simulink model "Huginn"  (R2024b)
settings: Solver=FixedStepAuto  StartTime=0.0  StopTime=525  FixedStep=0.1  RelTol=1e-3
model workspace (MAT data in the model file):
  N_P0 = 3
  fuel_map = [8.33e-06 8.33e-06 8.33e-06 8.33e-06 8.33e-06 8.33e-06 8.33e-06 8.33e-06 8.33e-06 8.33e-06 8.33e-06 8.33e-06 ... (2082 elements, 1041x2)]
  rpm_bp = [0 10 20 30 40 50 60 70 80 90 100 110 ... (671 elements, 671x1)]
  rpm_bp_fuel = [1200 1210 1220 1230 1240 1250 1260 1270 1280 1290 1300 1310 ... (1041 elements, 1041x1)]
  throttle_bp = [0 10 20 30 40 50 60 70 80 90 100]
  throttle_bp_fuel = [0; 1]
  torque_bp = [0.332105118453 0.337426322834 0.342845115066 0.348363542915 0.353983594259 0.359707194633 0.36553620448 0.371483133692 0.377549913828 0.383738457661 0.390050655328 0.396488370473 ... (901 elements, 901x1)]
  torque_map = [0 0 0 0 0 0 0 0 0 0 0 0 ... (7381 elements, 671x11)]
values from neighbouring files (symbols this model uses):
  rpm_fine = [1200 1210 1220 1230 1240 1250 1260 1270 1280 1290 1300 1310 ... (1041 elements, 1041x1)]    [optimised workspace.mat]    (also in run_before_huginn.m = (min(rpm_bp) : 10 : max(rpm_bp))')
  throttle_fine = [0 1]    [optimised workspace.mat]    (also in run_before_huginn.m = (min(throttle_bp) : 1 : max(throttle_bp))')
  throttle_profile = [14.9858312924 0 60 60 60 0.55631746946 8.17065947955 1.9881415447 9.75633320207 0.0428601079869 58.2417871472 60 ... (25 elements, 1x25)]    [Optimised_fuel_2.mat]    (also in optimised workspace.mat = [65.5401746966 57.4724229506 57.2057862197 67.539022656 57.9; other optmised.mat)
undefined symbols (not defined in the file or in its folder): DiscIntNeverNeededParam, dspblkCoreblockFVToolHelper, gcbh
(part 2 of 2)

== matlab function Huginn/Gear ==
  data: rpm input; rpm_out output; gear input; hold_timer input; g1 input; g2 input; g3 input; g4 input; up input; dn input; gear_out output; hold_out output; check output
function [rpm_out, gear_out, hold_out, check] = GearChange(rpm, gear, hold_timer, g1, g2, g3, g4, up, dn)
    ratios     = [g1, g2, g3, g4];
    num_gears  = numel(ratios);
    hysteresis = 0;   % increased from 150
    min_hold   = 20;
    check = 0; % 5 seconds at 0.1s timestep — increased from 20
    
    if hold_timer > 0
        rpm_out  = rpm;
        gear_out = double(gear);
        hold_out = hold_timer - 1;
    elseif rpm < (dn - hysteresis) && gear > 1
        rpm_out  = (ratios(gear-1) * rpm) / ratios(gear);
        gear_out = double(gear - 1);
        hold_out = min_hold;
    elseif rpm > (up + hysteresis) && gear < num_gears
        rpm_out  = (ratios(gear+1) * rpm) / ratios(gear);
        gear_out = double(gear + 1);
        hold_out = min_hold;
    else
        rpm_out  = rpm;
        gear_out = double(gear);
        hold_out = 0;
    end
    check = check + 1;
end

== matlab function Huginn/Total Acceleration ==
  data: accel input; total_accel output; neg_acceleration input
function total_accel = blk_accelTotal(accel, neg_acceleration)
    total_accel = accel + neg_acceleration;
end

== matlab function Huginn/Speed To RPM ==
  data: final_speed_ms input; rpm output; gear input; g1 input; g2 input; g3 input; g4 input; diff_red input; wheel_radius input
function rpm = blk_finalSpeedToRpm( ...
        final_speed_ms, gear, g1, g2, g3, g4, diff_red, wheel_radius)
    gear_ratios    = [g1, g2, g3, g4];
    gear_ratio     = gear_ratios(gear);
    combined_ratio = gear_ratio * diff_red;
    rpm = (final_speed_ms * combined_ratio * 60) / (2 * pi * wheel_radius);
end

== matlab function Huginn/MATLAB Function1 ==
  data: corr_torque input; accel output; wheel_radius input; mass input
function accel = AccelerationCalc(corr_torque, wheel_radius, mass)
    accel = (corr_torque * 1.38) / (mass * wheel_radius);
end

== matlab function Huginn/Has Ended ==
  data: distance_covered input; has_ended output; dist input
function has_ended = blk_hasEndedBasic(distance_covered, dist)
    has_ended = uint8(distance_covered >= dist);
end

== matlab function Huginn/MATLAB Function ==
  data: current_rpm input; torque output; rpm_bp input; torque_bp input
function torque = blk_getInterpolatedTorque(current_rpm, rpm_bp, torque_bp)
    % Offset carried over from original Python — review vs calibration
    torque_bp_adj = torque_bp + 70;
    torque = interp1(rpm_bp, torque_bp_adj, current_rpm, 'linear', 'extrap');
    torque = torque - 70;
end

== matlab function Huginn/drag ==
  data: init_speed_ms input; drag_force output; drag_coeff input; frontal_area input; mass input; air_density input; drag_accel output
function [drag_force, drag_accel] = blk_dragEffect( ...
        init_speed_ms, drag_coeff, frontal_area, mass, air_density)
    drag_force = 0.5 * drag_coeff * frontal_area * init_speed_ms^2 * air_density ;
    drag_accel = drag_force / mass;
end

== matlab function Huginn/Torque1 ==
  data: torque input; wheel_torque output; gear input; g1 input; g2 input; g3 input; g4 input; prim_red input; sec_red input; diff_red input; eta input
function wheel_torque  = TorqueGearRatio(torque, gear, g1, g2, g3, g4, ...
                                           prim_red, sec_red, diff_red, eta)
    ratios      = [g1, g2, g3, g4];
    gear_ratio  = ratios(gear);
    wheel_torque = torque * prim_red * sec_red * gear_ratio * eta * diff_red;
end

== matlab function Huginn/speed Calculator ==
  data: rpm input; init_speed_ms output; gear input; g1 input; g2 input; g3 input; g4 input; diff_red input; wheel_radius input; speed_kmh output
function [init_speed_ms, speed_kmh] = blk_speedCalc( ...
        rpm, gear, g1, g2, g3, g4, diff_red, wheel_radius)
    gear_ratios    = [g1, g2, g3, g4];
    gear_ratio     = gear_ratios(gear);
    combined_ratio = gear_ratio * diff_red;
    init_speed_ms  = (rpm * 2 * pi * wheel_radius) / (60 * combined_ratio);
    speed_kmh      = init_speed_ms * 3.6;
end

== matlab function Huginn/Total Deceleration ==
  data: tire_coeff input; neg_acceleration output; g input; drag_accel input
function neg_acceleration  = blk_decelerationCalc(tire_coeff, g, drag_accel)
    neg_acceleration = -(3.2* (tire_coeff * g)) - (1.8 * drag_accel);
end

== matlab function Huginn/Torque ==
  data: torque input; wheel_torque output; gear input; g1 input; g2 input; g3 input; g4 input; prim_red input; sec_red input; diff_red input; eta input
function wheel_torque  = TorqueGearRatio(torque, gear, g1, g2, g3, g4, ...
                                           prim_red, sec_red, diff_red, eta)
    ratios      = [g1, g2, g3, g4];
    gear_ratio  = ratios(gear);
    wheel_torque = torque * prim_red * sec_red * gear_ratio * eta * diff_red;
end

== matlab function Huginn/speed update ==
  data: init_speed_ms input; final_speed_ms output; total_accel input; time_step input
function final_speed_ms = SpeedUpdate(init_speed_ms, total_accel, time_step)
    final_speed_ms = init_speed_ms + (total_accel * time_step);
    if final_speed_ms < 0
        final_speed_ms = 0;
    end
end

== matlab function Huginn/Distance calculation ==
  data: init_speed_ms input; delta_distance output; final_speed_ms input; time_step input
function delta_distance = blk_distancePerTime( ...
        init_speed_ms, final_speed_ms, time_step)
    delta_distance = ((init_speed_ms + final_speed_ms) / 2) * time_step;
end
